simulink model "wavestarSimulator_2021a"  (R2021a)
settings: Solver=ode4  StartTime=0.0  StopTime=t_end  FixedStep=dt  RelTol=1e-3
values from neighbouring files (symbols this model uses):
  dt = 0.01    [rundown.m]    (also in wavestarMain.m)
  F2V_model = F2V.F2V_model_p    [wavestarMain.m]
  K_PI = tf(k_P) + tf(k_I, [1 0])    [wavestarMain.m]
libraries: simulink_extras x2
settings Model: Creator=Nicolas  LastModifiedBy=compu
settings DebuggingCC: UnconnectedInputMsg=none  UnconnectedOutputMsg=none  UnconnectedLineMsg=none
settings ModelReferenceCC: EnableRefExpFcnMdlSchedulingChecks=off
settings RTWCC: Description=Generic Real-Time Target  DLArmComputeVersion=20.02.1

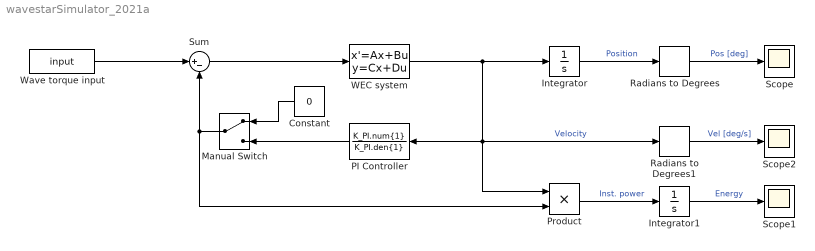
== system wavestarSimulator_2021a ==
  Constant : Constant  Value=0
  Integrator : Integrator
  Integrator1 : Integrator
  Manual Switch : ManualSwitch
  PI Controller : TransferFcn  Numerator=K_PI.num{1}  Denominator=K_PI.den{1}
  Product : Product
  Radians to Degrees : simulink_extras/Transformations/Radians to Degrees
  Radians to Degrees1 : simulink_extras/Transformations/Radians to Degrees
  Scope : Scope
  Scope1 : Scope
  Scope2 : Scope
  Sum : Sum  Inputs=|+-
  WEC system : StateSpace  A=F2V_model.A  B=F2V_model.B  C=F2V_model.C  D=F2V_model.D  InitialCondition=0
  Wave torque input : FromWorkspace  VariableName=input  SampleTime=dt  OutputAfterFinalValue=Setting to zero
  wires:
  Wave torque input/1 -> Sum/1
  Sum/1 -> WEC system/1
  WEC system/1 -> PI Controller/1, Product/1, Radians to Degrees1/1, Integrator/1  "Velocity"
  PI Controller/1 -> Manual Switch/2
  Manual Switch/1 -> Product/2, Sum/2
  Constant/1 -> Manual Switch/1
  Integrator/1 -> Radians to Degrees/1  "Position"
  Radians to Degrees/1 -> Scope/1  "Pos [deg]"
  Product/1 -> Integrator1/1  "Inst. power"
  Integrator1/1 -> Scope1/1  "Energy"
  Radians to Degrees1/1 -> Scope2/1  "Vel [deg/s]"
